simulink model "playback_data"  (R2015a)
settings: Solver=FixedStepDiscrete  SolverMode=SingleTasking  StartTime=76  StopTime=110  FixedStep=sample_time  RelTol=1e-3
undefined symbols (not defined in the file): A1_notch_f1, A2_notch_f1, A_kalman_swing_load, A_kalman_transverse, A_kalman_vertical, A_lpf_accelerometer, A_lpf_dtau, A_lpf_fourbar_angles, A_lpf_imu, A_lpf_lateral_angle, B1_lpf_accelerometer, B1_lpf_dtau, B1_lpf_fourbar_angles, B1_lpf_imu, B1_lpf_lateral_angle, B1_notch_f1, B2_lpf_accelerometer, B2_lpf_dtau, B2_lpf_fourbar_angles, B2_lpf_imu, B2_lpf_lateral_angle, B2_notch_f1, B_dx_versus_x0, B_kalman_swing_load, B_kalman_transverse, B_kalman_vertical, backwards_K_sag_of_t, backwards_P_sag_of_t, C_kalman_swing_load, C_kalman_transverse, C_kalman_vertical, com_leg_motor, com_torso, contact_threshold, control_start_time, d_ankle_to_foot, d_vertical_com, desired_com_forward_velocity, desired_com_lateral_velocity, desired_initial_leg_roll_left, desired_initial_leg_roll_right, desired_stance_beta2, desired_standing_torso_pitch, desired_standing_torso_roll, desired_standing_z, desired_torso_pitch, desired_torso_roll, Discrete, enable_bouncing, fcut_contact, fdesignblkfcn, forward_dx_of_dxstar, forward_x_of_dxstar, g, gcbh, HIP_MTR_MAX_CONT_TORQUE, HIP_MTR_MAX_TORQUE, i_leg_motor, i_robot, i_torso ... (+78)
libraries: simulink x65, dsparch4 x18, ctrlSharedLib x14, dspfdesign x4
(part 9 of 13)

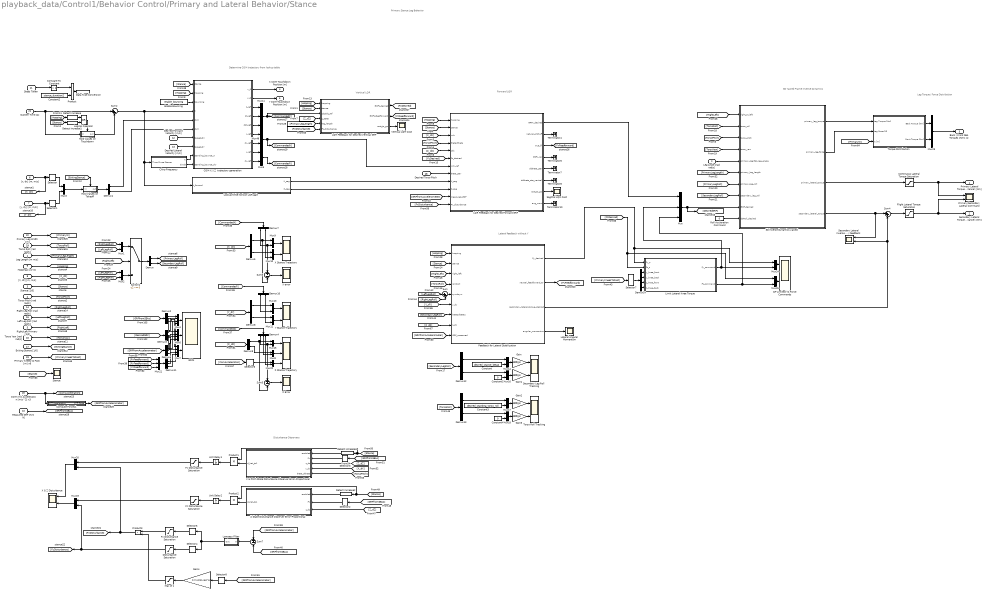
== system playback_data/Control1/Behavior Control/Primary and Lateral Behavior/Stance ==
  note: Lateral feedback without Y
  note: 3D Yawed Frame Inverse Dynamics
  note: Forward LQR
  note: Vertical LQR
  note: Determine COM trajectory
      | from lookup table
  note: Primary Stance Leg Behavior
  note: Disturbance Observers
  note: Leg Torque / Force
      | Distribution
  Leg Length [m m/s] : Inport
  Torso Pitch [rad rad/s] : Inport  Port=2
  Stance [1/0] : Inport  Port=3
  Leg Angle [rad rad/s] : Inport  Port=4
  Right/Left Primary [1/0] : Inport  Port=5
  "[x, dx] [m, m/s]" : Inport  Port=6
  "[y, dy] [m, m/s]" : Inport  Port=7
  "[z, dz] [m, m/s]" : Inport  Port=8
  Hopping [1 or 0] : Inport  Port=9
  Measured GRF [N N N] : Inport  Port=10
  Steps Taken : Inport  Port=11
  Desired Forward Velocity [m/s] : Inport  Port=12
  Desired Lateral Velocity [m/s] : Inport  Port=13
  Right Leg Roll [rad rad/s] : Inport  Port=14
  Left Leg Roll [rad rad/s] : Inport  Port=15
  Torso Yaw [rad rad/s] : Inport  Port=16
  Exiting Stance [1/0] : Inport  Port=17
  Desired Torso Pitch : Inport  Port=18
  Torso Roll [rad rad/s] : Inport  Port=19
  COM XYZ Acceleration [m/s^2] x3 : Inport  Port=20
  System Time [s] : Inport  Port=21
  Primary Leg Width [m] : Inport  Port=22
  Primary Knees to Foot [m] x6 : Inport  Port=23
  3D Inverse Dynamics yawed : MATLAB Function  TreatAsAtomicUnit=on
  COM X,Y,Z  trajectory generation : MATLAB Function  TreatAsAtomicUnit=on
  Chirp Frequency : Subsystem
  Compare To Constant : simulink/Logic and Bit Operations/Compare To Constant  relop=<  const=1  OutDataTypeStr=uint8
  Compute Forces1 : Subsystem
  Constant : Constant  Value=desired_stance_beta2
  Constant1 : Constant  Value=0
  Constant2 : Constant  Value=stance_duration/2
  Constant3 : Constant  Value=desired_standing_torso_roll
  Constant4 : Constant  Value=0
  Continuous Lateral Torque Saturation : Saturate  UpperLimit=max_primary_lateral_stance_torque  LowerLimit=-max_primary_lateral_stance_torque
      settings: AttributesFormatString=Top: %<UpperLimit>\nBottom: %<LowerLimit>
  Data Type Conversion : DataTypeConversion  OutDataTypeStr=double
  Demux{,1,5,7..10,12..13} (9 alike) : Demux  Outputs=2
  Demux{2..4,6,11} (5 alike) : Demux  Outputs=3
  Demux14 : Demux
  Detect Increase{,1..3} (4 alike) : simulink/Logic and Bit Operations/Detect Increase  vinit=0.0  InputProcessing=Inherited  OutDataTypeStr=boolean
  "Disturbance Saturation " : Saturate  UpperLimit=100  LowerLimit=-100
      settings: AttributesFormatString=Top: %<UpperLimit>\nBottom: %<LowerLimit>
  Enable Bouncing : Constant  Value=enable_bouncing  SampleTime=sample_time
  Feedback for Lateral Stabilization : MATLAB Function  TreatAsAtomicUnit=on
  Flight Lateral Torque Saturation : Saturate  UpperLimit=HIP_MTR_MAX_CONT_TORQUE  LowerLimit=-HIP_MTR_MAX_CONT_TORQUE
      settings: AttributesFormatString=Top: %<UpperLimit>\nBottom: %<LowerLimit>
  Fx Disturbance Saturation : Saturate  UpperLimit=100  LowerLimit=-100
      settings: AttributesFormatString=Top: %<UpperLimit>\nBottom: %<LowerLimit>
  "Fx Disturbance Saturation " : Saturate  UpperLimit=100  LowerLimit=-100
      settings: AttributesFormatString=Top: %<UpperLimit>\nBottom: %<LowerLimit>
  Fz Disturbance Saturation : Saturate  UpperLimit=100  LowerLimit=-100
      settings: AttributesFormatString=Top: %<UpperLimit>\nBottom: %<LowerLimit>
  GRFs : Scope  NumInputPorts=3
      settings: TimeRange=37.999  YMin=-1250~-2000~-1250  YMax=1500~3750~1750  SampleInput=on
  Gain{,1..3} (4 alike) : Gain  Gain=180/pi
  Gain4 : Gain  Gain=2/(m_total_real*g)
  Hold Values on Takeoff : Subsystem
  Hold Values on Touchdown : Subsystem
  LQR Feedback for Desired Forward GRF : MATLAB Function  TreatAsAtomicUnit=on
  LQR Feedback for Desired Vertical GRF : MATLAB Function  TreatAsAtomicUnit=on
  Lateral Angular Momentum : Scope
      settings: YMin=-3.5  YMax=4  SaveName=ScopeData20  SampleInput=on
  Limit Lateral Knee Torque : MATLAB Function  TreatAsAtomicUnit=on
  Logical Operator : Logic  Operator=OR  AllPortsSameDT=off  OutDataTypeStr=boolean
  Lookup finite horizon LQR gain : MATLAB Function  TreatAsAtomicUnit=on
  Lowpass Filter : Subsystem  DialogController=fdesignblkfcn  InitFcn=fdesignblkfcn(gcbh, {'InitFcn'});  mask(Lowpass Filter){}
      mask help: Design a lowpass filter
      settings: CopyFcn=fdesignblkfcn(gcbh, {'CopyFcn'});
      mask Help: helpview(mapfilelocation('dsp'), 'dsplowpassfilter');
      mask Display: disp('Lowpass')
  Max of 1 : Saturate  UpperLimit=1  LowerLimit=0
      settings: AttributesFormatString=Top: %<UpperLimit>\nBottom: %<LowerLimit>
  Mux : Mux  Inputs=3
  Mux{1..3,5,8..10,12..20,22..25,49} (21 alike) : Mux  Inputs=2
  Mux11 : Mux  Inputs=3
  Mux21 : Mux  Inputs=3
  Mux4 : Mux
  Mux6 : Mux
  Mux7 : Mux
  Primary/Secondary Lateral Command : Scope  NumInputPorts=2
      settings: YMin=40~-5  YMax=150~5  SaveName=ScopeData25  SampleInput=on
  Product{,1..3} (4 alike) : Product
  QP Limited YZ Force Commands : Scope  NumInputPorts=2
      settings: YMin=-200~0  YMax=30~700  SaveName=ScopeData26  SampleInput=on
  Roll Accleration Command : Constant  Value=0
  Sagittal LQR Cost : Scope
      settings: YMin=22.5  YMax=62.5  SaveName=ScopeData10  SampleInput=on
  Secondary Lateral Inverse Dynamics / Feedback : Scope  NumInputPorts=2
      settings: YMin=-3.5~-5  YMax=4~5  SaveName=ScopeData9  SampleInput=on
  Secondary Leg Roll Tracking : Scope  NumInputPorts=2
      settings: YMin=-3.5~-5  YMax=4~5  SaveName=ScopeData12  SampleInput=on
  Selector : Selector  InputPortWidth=2  Indices=[2]
  Selector1 : Selector  InputPortWidth=2  Indices=[2]
  Selector{2,4,6,8} (4 alike) : Selector  InputPortWidth=3  Indices=[3]
  Selector3 : Selector  InputPortWidth=3  Indices=[1]
  Selector5 : Selector  InputPortWidth=3  Indices=[1]
  Selector7 : Selector  InputPortWidth=6  Indices=[2 5 3 6]
  Stance : Scope
      settings: YMin=-0.05  YMax=0.11  SaveName=stance_time_history  SampleInput=on
  Sum : Sum  Inputs=|+-
  Sum2 : Sum  Inputs=|+-
  Sum4 : Sum  Inputs=|++
  Sum5 : Sum  Inputs=+-
  Sum6 : Sum  Inputs=+-
  Sum7 : Sum  Inputs=+-
  Switch1 : Switch  Criteria=u2 ~= 0
  Terminator{4,6..8,10} (5 alike) : Terminator
  Torque Distribution : Subsystem
  Torso Roll Tracking : Scope  NumInputPorts=2
      settings: YMin=-3.5~-5  YMax=4~5  SaveName=ScopeData15  SampleInput=on
  Unit Delay1 : UnitDelay  SampleTime=sample_time
  Unit Delay2 : UnitDelay  SampleTime=sample_time
  Vertical LQR Cost : Scope
      settings: YMin=11  YMax=16  SaveName=ScopeData18  SampleInput=on
  X & Pitch State Disturbance Observer Error-Proportional : MATLAB Function  TreatAsAtomicUnit=on
  X & Z Disturbance : Scope  NumInputPorts=2
      settings: YMin=-125~-800  YMax=175~700  SaveName=ScopeData16  SampleInput=on
  X Stance Trajectory : Scope  NumInputPorts=2
      settings: YMin=0~-0.02  YMax=0.005~0.03  SaveName=ScopeData8  SampleInput=on
  X error : Scope
      settings: YMin=-0.05  YMax=0.11  SaveName=ScopeData24  SampleInput=on
  Y Stance Trajectory : Scope  NumInputPorts=2
      settings: YMin=0.005~-0.5  YMax=0.1~0.3  SaveName=ScopeData5  SampleInput=on
  Z Error : Scope
      settings: YMin=-0.007  YMax=0.0005  SaveName=ScopeData23  SampleInput=on
  Z Stance Trajectory : Scope  NumInputPorts=3
      settings: YMin=0.85~-0.4~-3  YMax=0.98~0.6~11  SaveName=z_stance_trajectory  SampleInput=on
  Z State Disturbance Observer Error-Proportional : MATLAB Function  TreatAsAtomicUnit=on
  Primary Lateral Torque Command (stance) [Nm] : Outport
  Secondary Lateral Torque Command (stance) [Nm] : Outport  Port=2
  Back / Front SEA Torques [Nm] x2 : Outport  Port=3
  X COM Touchdown Position [m] : Outport  Port=4
  Y COM Touchdown Position [m] : Outport  Port=5
  wires:
  Fz Disturbance Saturation/1 -> Mux19/1
  Selector5/1 -> "Fx Disturbance Saturation "/1
  "Disturbance Saturation "/1 -> [FzDisturbance], Mux19/2
  Max of 1/1 -> Product3/2
  "Fx Disturbance Saturation "/1 -> Product3/1
  Gain4/1 -> Max of 1/1
  Selector8/1 -> Gain4/1
  [GRFfromAccelerometer] -> Selector8/1
  Limit Lateral Knee Torque/2(Fz_command) -> Mux/3, Mux25/2
  [FzDisturbance] -> LQR Feedback for Desired Vertical GRF/6(Fz_disturbance)
  [FxDisturbance] -> LQR Feedback for Desired Forward GRF/12(Fx_disturbance)
  Lowpass Filter/1(Out) -> Selector5/1, Selector4/1
  Chirp Frequency/2(dw/dt) -> COM X,Y,Z  trajectory generation/10(standing_bounce_dw)
  [Stance] -> Stance/1
  Chirp Frequency/1(w) -> COM X,Y,Z  trajectory generation/9(standing_bounce_w)
  Selector2/1 -> Z State Disturbance Observer Error-Proportional/2(Fz)
  Sum7/1 -> Lowpass Filter/1(In)
  Product3/1 -> Mux20/2, [FxDisturbance]
  Mux20/1 -> X & Z Disturbance/1
  [GRFfromAccelerometer] -> Sum7/1
  Sum6/1 -> X error/1
  Demux7/1 -> Mux9/2, Sum6/1
  Demux5/1 -> Mux9/1, Sum6/2
  Unit Delay2/1 -> Fz Disturbance Saturation/1
  Unit Delay1/1 -> Fx Disturbance Saturation/1
  Selector3/1 -> X & Pitch State Disturbance Observer Error-Proportional/2(Fx)
  Fx Disturbance Saturation/1 -> Mux20/1
  Enable Bouncing/1 -> COM X,Y,Z  trajectory generation/3(bouncing)
  [RightLeft] -> Feedback for Lateral Stabilization/3(right_left)
  Constant4/1 -> Mux18/2
  Mux18/1 -> Gain3/1
  Demux13/2 -> Mux18/1
  Constant3/1 -> Mux17/2
  Demux13/1 -> Mux17/1
  Mux17/1 -> Gain2/1
  Gain3/1 -> Torso Roll Tracking/2
  Gain2/1 -> Torso Roll Tracking/1
  [TorsoRoll] -> Demux13/1
  Constant1/1 -> Mux16/2
  Demux12/2 -> Mux16/1
  Mux16/1 -> Gain1/1
  Gain1/1 -> Secondary Leg Roll Tracking/2
  Gain/1 -> Secondary Leg Roll Tracking/1
  Constant/1 -> Mux14/2
  Demux12/1 -> Mux14/1
  Mux14/1 -> Gain/1
  [SecondaryLegRoll] -> Demux12/1
  Feedback for Lateral Stabilization/3(secondary_lateral_torque_desired) -> Sum4/2, Secondary Lateral Inverse Dynamics / Feedback/2
  Sum4/1 -> Flight Lateral Torque Saturation/1
  3D Inverse Dynamics yawed/3(primary_lateral_torque) -> Continuous Lateral Torque Saturation/1
  3D Inverse Dynamics yawed/4(secondary_lateral_torque) -> Secondary Lateral Inverse Dynamics / Feedback/1, Sum4/1
  Sum/1 -> Feedback for Lateral Stabilization/5(symdsym)
  [SecondaryLegRoll] -> Feedback for Lateral Stabilization/7(beta2dbeta2)
  [Y_dY] -> Feedback for Lateral Stabilization/6(y_dy)
  [RightLegRoll] -> Sum/2
  [LeftLegRoll] -> Sum/1
  Roll Accleration Command/1 -> 3D Inverse Dynamics yawed/10(ddRoll_desired)
  Feedback for Lateral Stabilization/1(Fy_desired) -> Limit Lateral Knee Torque/1(Fy_s), Mux24/1
  Continuous Lateral Torque Saturation/1 -> Primary/Secondary Lateral Command/1, Primary Lateral Torque Command (stance) [Nm]/1
  Demux11/3 -> Mux7/4
  Demux11/2 -> Mux6/4
  Demux11/1 -> Mux4/4
  Mux/1 -> [DesiredGRF], 3D Inverse Dynamics yawed/9(GRF_desired)
  LQR Feedback for Desired Forward GRF/1(GRFx_desired) -> Mux/1
  Left Leg Roll [rad rad/s]/1 -> [LeftLegRoll]
  Right/Left Primary [1/0]/1 -> [RightLeft]
  [CommandedY] -> Demux10/1
  [CommandedX] -> Demux7/1
  [Y_dY] -> Demux8/1
  Demux10/2 -> Mux12/2
  Demux10/1 -> Mux13/2
  Demux8/2 -> Mux12/1
  Demux8/1 -> Mux13/1
  Mux12/1 -> Y Stance Trajectory/2
  Mux13/1 -> Y Stance Trajectory/1
  [X_dX] -> Demux5/1
  Demux7/2 -> Mux10/2
  Demux5/2 -> Mux10/1
  Mux10/1 -> X Stance Trajectory/2
  Mux9/1 -> X Stance Trajectory/1
  Demux3/3 -> Mux7/2
  Demux3/2 -> Mux6/2
  Demux3/1 -> Mux4/2
  Demux2/3 -> Mux7/1
  Demux2/2 -> Mux6/1
  Mux7/1 -> GRFs/3
  Mux6/1 -> GRFs/2
  Demux2/1 -> Mux4/1
  Mux4/1 -> GRFs/1
  [DesiredGRF] -> Demux3/1
  [GRFfromSEAs] -> Demux2/1
  Torso Roll [rad rad/s]/1 -> [TorsoRoll]
  [PrimaryLegLength] -> LQR Feedback for Desired Vertical GRF/5(leg_length)
  Leg Length [m m/s]/1 -> [PrimaryLegLength]
  System Time [s]/1 -> Sum2/1, Hold Values on Touchdown/1(in)
  [GRFfromAccelerometer] -> Feedback for Lateral Stabilization/9(GRF_measured)
  [Hopping] -> Feedback for Lateral Stabilization/1(hopping)
  [ExitingStance] -> Hold Values on Takeoff/Trigger
  Exiting Stance [1/0]/1 -> [ExitingStance]
  Torso Yaw [rad rad/s]/1 -> [TorsoYaw]
  Desired Lateral Velocity [m/s]/1 -> COM X,Y,Z  trajectory generation/8(target_DY)
  Selector1/1 -> Mux3/2
  Hold Values on Takeoff/1(out) -> Demux1/1
  Mux3/1 -> Hold Values on Takeoff/1(in)
  "[y, dy] [m, m/s]"/1 -> Selector1/1, [Y_dY]
  [RightLeft] -> Switch1/2
  [RightLegRoll] -> Mux2/2
  [LeftLegRoll] -> Mux2/1
  [LeftLegRoll] -> Mux1/2
  [RightLegRoll] -> Mux1/1
  Right Leg Roll [rad rad/s]/1 -> [RightLegRoll]
  Mux2/1 -> Switch1/3
  Mux1/1 -> Switch1/1
  Demux/1 -> [PrimaryLegRoll]
  Demux/2 -> [SecondaryLegRoll]
  Switch1/1 -> Demux/1
  [PrimaryLegRoll] -> 3D Inverse Dynamics yawed/7(primary_leg_roll)
  [SecondaryLegRoll] -> 3D Inverse Dynamics yawed/8(secondary_leg_roll)
  Leg Angle [rad rad/s]/1 -> 3D Inverse Dynamics yawed/5(primary_sagittal_leg_angle)
  [PrimaryLegLength] -> 3D Inverse Dynamics yawed/6(primary_leg_length)
  [TorsoYaw] -> 3D Inverse Dynamics yawed/4(torso_yaw)
  [TorsoRoll] -> 3D Inverse Dynamics yawed/2(torso_roll)
  [TorsoPitch] -> 3D Inverse Dynamics yawed/3(torso_pitch)
  Mux5/1 -> [CommandedY]
  COM X,Y,Z  trajectory generation/2(y_0) -> Y COM Touchdown Position [m]/1
  [TorsoRoll] -> Feedback for Lateral Stabilization/4(rolldroll)
  [Stance] -> Feedback for Lateral Stabilization/2(stance)
  [Hopping] -> LQR Feedback for Desired Vertical GRF/1(hopping)
  Selector/1 -> Mux3/1
  Demux1/1 -> COM X,Y,Z  trajectory generation/5(dx0)
  [Stance] -> Detect Increase1/1
  [Hopping] -> Detect Increase/1
  Compare To Constant/1 -> Product/1
  Detect Increase1/1 -> Logical Operator/2
  Detect Increase/1 -> Logical Operator/1
  Constant2/1 -> Product/2
  Product/1 -> Data Type Conversion/1
  Steps Taken/1 -> Compare To Constant/1
  [GRFfromAccelerometer] -> LQR Feedback for Desired Forward GRF/11(measured_GRF)
  Measured GRF [N N N]/1 -> [GRFfromSEAs]
  [Hopping] -> LQR Feedback for Desired Forward GRF/1(hopping)
  [Hopping] -> COM X,Y,Z  trajectory generation/2(hopping)
  Hopping [1 or 0]/1 -> [Hopping]
  [RightLeft] -> 3D Inverse Dynamics yawed/1(right_or_left)
  Torso Pitch [rad rad/s]/1 -> [TorsoPitch]
  LQR Feedback for Desired Forward GRF/8(ang_mom) -> Terminator10/1
  LQR Feedback for Desired Forward GRF/7(cost_to_go) -> Sagittal LQR Cost/1
  LQR Feedback for Desired Forward GRF/6(ddtheta_star_neutral) -> Terminator8/1
  LQR Feedback for Desired Forward GRF/5(ddtheta_star) -> Terminator7/1
  LQR Feedback for Desired Vertical GRF/3(cost_to_go) -> Vertical LQR Cost/1
  Demux1/2 -> COM X,Y,Z  trajectory generation/6(dy0)
  "[x, dx] [m, m/s]"/1 -> Selector/1, [X_dX]
  Logical Operator/1 -> Hold Values on Touchdown/Trigger
  [Stance] -> LQR Feedback for Desired Vertical GRF/2(stance)
  Stance [1/0]/1 -> [Stance]
  Hold Values on Touchdown/1(out) -> Sum2/2
  LQR Feedback for Desired Vertical GRF/1(GRFz_desired) -> [FzDesired]
  Sum2/1 -> Chirp Frequency/1(Time Since Stance), Lookup finite horizon LQR gain/1(t_forward), COM X,Y,Z  trajectory generation/4(t)
  Desired Forward Velocity [m/s]/1 -> COM X,Y,Z  trajectory generation/7(target_DX)
  [Z_dZ] -> LQR Feedback for Desired Forward GRF/5(zdz)
  Lookup finite horizon LQR gain/1(K_sag) -> LQR Feedback for Desired Forward GRF/9(K_sag)
  Desired Torso Pitch/1 -> LQR Feedback for Desired Forward GRF/8(theta_star)
  Mux49/1 -> LQR Feedback for Desired Forward GRF/7(xdx_ref), [CommandedX]
  [TorsoPitch] -> LQR Feedback for Desired Forward GRF/4(thetadtheta)
  [X_dX] -> LQR Feedback for Desired Forward GRF/3(xdx)
  Mux11/1 -> LQR Feedback for Desired Vertical GRF/3(zdzddz_ref), [CommandedZ]
  COM X,Y,Z  trajectory generation/5(ddz_ref) -> Mux11/3
  COM X,Y,Z  trajectory generation/4(dz_ref) -> Mux11/2
  COM X,Y,Z  trajectory generation/1(x_0) -> X COM Touchdown Position [m]/1
  COM X,Y,Z  trajectory generation/9(dy_ref) -> Mux5/2
  COM X,Y,Z  trajectory generation/8(y_ref) -> Mux5/1
  COM X,Y,Z  trajectory generation/7(dx_ref) -> Mux49/2
  COM X,Y,Z  trajectory generation/6(x_ref) -> Mux49/1
  [Stance] -> LQR Feedback for Desired Forward GRF/2(stance)
  COM X,Y,Z  trajectory generation/3(z_ref) -> Mux11/1
  [Z_dZ] -> LQR Feedback for Desired Vertical GRF/4(z_state)
  Lookup finite horizon LQR gain/2(P_sag) -> LQR Feedback for Desired Forward GRF/10(P_sag)
  [Stance] -> COM X,Y,Z  trajectory generation/1(stance)
  LQR Feedback for Desired Forward GRF/4(GRFx_lqr) -> Terminator6/1
  Feedback for Lateral Stabilization/4(angular_momentum) -> Lateral Angular Momentum/1
  Demux6/1 -> Mux4/3
  Demux6/2 -> Mux6/3
  Demux6/3 -> Mux7/3
  Flight Lateral Torque Saturation/1 -> Primary/Secondary Lateral Command/2, Secondary Lateral Torque Command (stance) [Nm]/1
  "[z, dz] [m, m/s]"/1 -> [Z_dZ]
  [Z_dZ] -> X & Pitch State Disturbance Observer Error-Proportional/3(z_dz)
  [TorsoPitch] -> X & Pitch State Disturbance Observer Error-Proportional/5(theta_dtheta)
  [X_dX] -> X & Pitch State Disturbance Observer Error-Proportional/4(x_dx)
  [GRFfromSEAs] -> Selector3/1
  Detect Increase3/1 -> X & Pitch State Disturbance Observer Error-Proportional/1(enabled)
  Detect Increase2/1 -> Z State Disturbance Observer Error-Proportional/1(enabled)
  [GRFfromSEAs] -> Selector2/1
  [Z_dZ] -> Z State Disturbance Observer Error-Proportional/3(z_dz)
  Product1/1 -> Unit Delay1/1
  Product2/1 -> Unit Delay2/1
  X & Pitch State Disturbance Observer Error-Proportional/1(d_hat_tp1) -> Product1/2
  [Stance] -> Product1/1, Detect Increase3/1
  Z State Disturbance Observer Error-Proportional/1(d_hat_tp1) -> Product2/2
  [Stance] -> Product2/1, Detect Increase2/1
  Mux19/1 -> X & Z Disturbance/2
  [GRFfromSEAs] -> Sum7/2
  Selector4/1 -> "Disturbance Saturation "/1
  COM XYZ Acceleration [m/s^2] x3/1 -> Compute Forces1/1(XYZ Acceleration), [ComAcceleration]
  [GRFfromAccelerometer] -> Demux6/1
  LQR Feedback for Desired Vertical GRF/2(GRFz_feedforward) -> [FzFeedforward]
  Mux21/1 -> Demux11/1
  [FzFeedforward] -> Mux21/3
  Mux15/1 -> Z Stance Trajectory/1
  Mux8/1 -> Z Stance Trajectory/2
  [Z_dZ] -> Demux9/1
  Demux9/1 -> Mux15/1, Sum5/2
  Demux9/2 -> Mux8/1
  Demux4/1 -> Mux15/2, Sum5/1
  Demux4/2 -> Mux8/2
  Demux4/3 -> Mux22/2
  [CommandedZ] -> Demux4/1
  Sum5/1 -> Z Error/1
  Mux22/1 -> Z Stance Trajectory/3
  [ComAcceleration] -> Selector6/1
  Selector6/1 -> Mux22/1
  3D Inverse Dynamics yawed/1(primary_leg_torque) -> Torque Distribution/1(Leg Torque [Nm])
  [PrimaryW] -> Torque Distribution/3(w [m])
  3D Inverse Dynamics yawed/2(primary_leg_force) -> Torque Distribution/2(Leg Force [N])
  Primary Leg Width [m]/1 -> [PrimaryW]
  Torque Distribution/1(Back Torque [Nm]) -> Mux23/1
  Torque Distribution/2(Front Torque [Nm]) -> Mux23/2
  Mux23/1 -> Back / Front SEA Torques [Nm] x2/1
  [FxFeedforward] -> Mux21/1
  [FzDesired] -> LQR Feedback for Desired Forward GRF/6(Fz_desired)
  [FzDesired] -> Limit Lateral Knee Torque/2(Fz_s), Mux25/1
  [Z_dZ] -> Feedback for Lateral Stabilization/8(z_dz)
  [FyFeedforward] -> Mux21/2
  Compute Forces1/1(XYZ Force) -> [GRFfromAccelerometer]
  LQR Feedback for Desired Forward GRF/3(true_ff) -> [FxFeedforward]
  LQR Feedback for Desired Forward GRF/2(netural_pitch_ff) -> Terminator4/1
  Feedback for Lateral Stabilization/2(neutral_feedforward_Fy) -> [FyFeedforward]
  Primary Knees to Foot [m] x6/1 -> [PrimaryKneesToFoot]
  [PrimaryKneesToFoot] -> Selector7/1
  Demux14/1 -> Limit Lateral Knee Torque/3(y_knee_front)
  Demux14/2 -> Limit Lateral Knee Torque/4(y_knee_back)
  Demux14/3 -> Limit Lateral Knee Torque/5(z_knee_front)
  Demux14/4 -> Limit Lateral Knee Torque/6(z_knee_back)
  Selector7/1 -> Demux14/1
  Mux24/1 -> QP Limited YZ Force Commands/1
  Mux25/1 -> QP Limited YZ Force Commands/2
  Limit Lateral Knee Torque/1(Fy_command) -> Mux24/2, Mux/2

== system playback_data/Control1/Behavior Control/Secondary Leg Behavior/Back//Front PD ==
  Desired Position [rad] [back front] : Inport
  Desired Velocity [rad/s] [back front] : Inport  Port=2
  Measured Position [rad] [back front] : Inport  Port=3
  Measured Velocity [rad/s] [back front] : Inport  Port=4
  Back Tracking : Scope  NumInputPorts=2
      settings: YMin=3.725~-1  YMax=4.05~0.9  SaveName=ScopeData6  SampleInput=on
  Front Tracking : Scope  NumInputPorts=2
      settings: YMin=-1~-0.8  YMax=1~1.4  SaveName=ScopeData31  SampleInput=on
  Kp_SEA_Trajectory : Constant  Value=kp_velocity_swing_trajectory
  Mux{1..2,12..13} (4 alike) : Mux  Inputs=2
  Product1 : Product
  Selector{,1..3} (4 alike) : Selector  InputPortWidth=2  Indices=[1]
  Selector{4..7} (4 alike) : Selector  InputPortWidth=2  Indices=[2]
  Sum7 : Sum  Inputs=|+-
  Sum9 : Sum
  Commanded Velocity [rad/s] [back front] : Outport
  wires:
  Selector7/1 -> Mux1/2
  Selector6/1 -> Mux1/1
  Selector4/1 -> Mux2/1
  Selector5/1 -> Mux2/2
  Selector3/1 -> Mux12/2
  Selector2/1 -> Mux12/1
  Selector1/1 -> Mux13/2
  Selector/1 -> Mux13/1
  Mux2/1 -> Front Tracking/1
  Mux1/1 -> Front Tracking/2
  Desired Position [rad] [back front]/1 -> Sum7/1, Selector1/1, Selector5/1
  Mux13/1 -> Back Tracking/1
  Mux12/1 -> Back Tracking/2
  Product1/1 -> Sum9/1
  Sum7/1 -> Product1/1
  Measured Position [rad] [back front]/1 -> Sum7/2, Selector/1, Selector4/1
  Desired Velocity [rad/s] [back front]/1 -> Sum9/2, Selector2/1, Selector6/1
  Measured Velocity [rad/s] [back front]/1 -> Selector3/1, Selector7/1
  Sum9/1 -> Commanded Velocity [rad/s] [back front]/1
  Kp_SEA_Trajectory/1 -> Product1/2

== system playback_data/Control1/Behavior Control/Secondary Leg Behavior/Lowpass Filter (Swing) ==
  In : Inport
  Generated Filter Block : dsparch4/Biquad Filter  Tag=BlockMethodSubSystem  IIRFiltStruct=Direct form II  CoeffSource=Specify via dialog  BiQuadCoeffs=[1.0218648663828083 -2 1.0218648663828083 1 -1.9114378222117407 0.91557643487411833]  a0Flag=Warning  IC=0  ICnum=0  ICden=0  denAccumFracLength=30  denProdOutputFracLength=30  secondMemoryFracLength=15  roundingMode=Floor  overflowMode=off  ScaleValues=[0.0041174265739107223;22.985401576126357]  optimizeScaleValues=off  ScaleValueMode=Specify via input port (g)  scaleValueFracLength=14  FilterSource=Specify via dialog  FilterObject=Hm_biquad
  Out : Outport
  wires:
  Generated Filter Block/1 -> Out/1
  In/1 -> Generated Filter Block/1

== system playback_data/Control1/Behavior Control/State Estimation/Kalman Filtering ==
  "COM from Left Foot [body, yawed, global]" : Inport  SampleTime=sample_time
  "COM from Right Foot [body, yawed, global]" : Inport  Port=2  SampleTime=sample_time
  GRFx [N] : Inport  Port=3  SampleTime=sample_time
  GRFy [N] : Inport  Port=4  SampleTime=sample_time
  GRFz [N] : Inport  Port=5  SampleTime=sample_time
  Right Vertical GRF [N] : Inport  Port=6  SampleTime=sample_time
  Left Vertical GRF [N] : Inport  Port=7  SampleTime=sample_time
  "Initial [x, dx, ddx] [m, m/s, m/s^2]" : Inport  Port=8  PortDimensions=3  SampleTime=sample_time
  "Initial [y, dy, ddy] [m, m/s, m/s^2]" : Inport  Port=9  PortDimensions=3  SampleTime=sample_time
  "Initial [z, dz, ddz] [m m/s m/s^2]" : Inport  Port=10  PortDimensions=3  SampleTime=sample_time
  COM XYZ Acceleration [m/s^2] x3 : Inport  Port=11  SampleTime=sample_time
  Entering Stance [1/0] : Inport  Port=12  PortDimensions=1  SampleTime=sample_time
  Enable : EnablePort  StatesWhenEnabling=reset
  Difference : simulink/Discrete/Difference  ICPrevInput=0.0  InputProcessing=Inherited  OutMin=[]  OutMax=[]  OutDataType=fixdt(1, 16)  OutScaling=2^-10  DoSatur=off
  Difference1 : simulink/Discrete/Difference  ICPrevInput=0.0  InputProcessing=Inherited  OutMin=[]  OutMax=[]  OutDataType=fixdt(1, 16)  OutScaling=2^-10  DoSatur=off
  Difference2 : simulink/Discrete/Difference  ICPrevInput=0.0  InputProcessing=Inherited  OutMin=[]  OutMax=[]  OutDataType=fixdt(1, 16)  OutScaling=2^-10  DoSatur=off
  Logical Operator : Logic  Operator=NOT  AllPortsSameDT=off  OutDataTypeStr=boolean
  Measurement Noise Covariance Matricies : MATLAB Function  TreatAsAtomicUnit=on
  Mux : Mux  Inputs=3
  Mux1 : Mux  Inputs=3
  Mux3 : Mux  Inputs=3
  P0_kalman_transverse : Constant  Value=P0_kalman_transverse
  P0_kalman_transverse1 : Constant  Value=P0_kalman_transverse
  P0_kalman_vertical : Constant  Value=P0_kalman_vertical
  Product : Product
  Product1 : Product
  Product2 : Product
  X State Kalman Filter : ctrlSharedLib/Kalman Filter  TimeDomain=Discrete-Time  UseCurrentEstimator=on  ModelSource=Individual A, B, C, D matrices  ModelSourceVariable=A_kf  A=A_kalman_transverse  B=B_kalman_transverse  C=C_kalman_transverse  D=0  NumberOfStates=2  NumberOfInputs=1  NumberOfOutputs=2  InitialEstimateSource=Input port  X0=initial_dx_estimate  P0=P0_kalman_transverse  UseK=off  UseGH=on  NumberOfProcessNoiseInputs=1  G=G_kalman_transverse  TimeInvariantG=on  H=0  TimeInvariantH=on  Q=Q_kalman_GRF_difference  TimeInvariantQ=on  R=1  TimeInvariantR=off  N=0  TimeInvariantN=on  AddInputPort=on  AddEnablePort=off  ExternalReset=Rising  OutputEstimatedY=off  OutputP=on  Ts=sample_time
  Y State Kalman Filter : ctrlSharedLib/Kalman Filter  TimeDomain=Discrete-Time  UseCurrentEstimator=on  ModelSource=Individual A, B, C, D matrices  ModelSourceVariable=A_kf  A=A_kalman_transverse  B=B_kalman_transverse  C=C_kalman_transverse  D=0  NumberOfStates=2  NumberOfInputs=1  NumberOfOutputs=2  InitialEstimateSource=Input port  X0=initial_dy_estimate  P0=P0_kalman_transverse  UseK=off  UseGH=on  NumberOfProcessNoiseInputs=1  G=G_kalman_transverse  TimeInvariantG=on  H=0  TimeInvariantH=on  Q=Q_kalman_GRF_difference  TimeInvariantQ=on  R=1  TimeInvariantR=off  N=0  TimeInvariantN=on  AddInputPort=on  AddEnablePort=off  ExternalReset=Rising  OutputEstimatedY=off  OutputP=on  Ts=sample_time
  Z State Kalman Filter : ctrlSharedLib/Kalman Filter  TimeDomain=Discrete-Time  UseCurrentEstimator=on  ModelSource=Individual A, B, C, D matrices  ModelSourceVariable=A_kf  A=A_kalman_vertical  B=B_kalman_vertical  C=C_kalman_vertical  D=0  NumberOfStates=2  NumberOfInputs=1  NumberOfOutputs=2  InitialEstimateSource=Input port  X0=[initial_z_estimate; initial_dz_estimate]  P0=P0_kalman_vertical  UseK=off  UseGH=on  NumberOfProcessNoiseInputs=1  G=G_kalman_vertical  TimeInvariantG=on  H=0  TimeInvariantH=on  Q=Q_kalman_GRF_difference  TimeInvariantQ=on  R=1  TimeInvariantR=off  N=0  TimeInvariantN=on  AddInputPort=on  AddEnablePort=off  OutputEstimatedY=off  OutputP=on  Ts=sample_time
  eigen values : MATLAB Function  TreatAsAtomicUnit=on
  eigen values1 : MATLAB Function  TreatAsAtomicUnit=on
  eigen values2 : MATLAB Function  TreatAsAtomicUnit=on
  left x yawed : Selector  InputPortWidth=9  Indices=[4]
  left y yawed : Selector  InputPortWidth=9  Indices=[5]
  left z yawed : Selector  InputPortWidth=9  Indices=[6]
  right x yawed : Selector  InputPortWidth=9  Indices=[4]
  right y yawed : Selector  InputPortWidth=9  Indices=[5]
  right z yawed : Selector  InputPortWidth=9  Indices=[6]
  x acceleration : Selector  InputPortWidth=3  Indices=[1]
  y acceleration : Selector  InputPortWidth=3  Indices=[2]
  z acceleration : Selector  InputPortWidth=3  Indices=[3]
  "[x, dx, ddx] [m/s, m/s^2]" : Outport
  "[y, dy, ddy] [m/s, m/s^2]" : Outport  Port=2
  "[z, dz, ddz] [m, m/s, m/s^2]" : Outport  Port=3
  "[x, dx, ddx] uncertainty" : Outport  Port=4
  "[y, dy, ddy] uncertainty" : Outport  Port=5
  "[z, dz, ddz] uncertainty" : Outport  Port=6
  wires:
  GRFz [N]/1 -> Difference/1
  Product/1 -> Z State Kalman Filter/1
  Product1/1 -> Y State Kalman Filter/1
  Product2/1 -> X State Kalman Filter/1
  Difference2/1 -> Product2/2
  Difference1/1 -> Product1/2
  Entering Stance [1/0]/1 -> Logical Operator/1, X State Kalman Filter/5, Y State Kalman Filter/5
  Difference/1 -> Product/2
  Logical Operator/1 -> Product1/1, Product/1, Product2/1
  eigen values/1(E) -> "[z, dz, ddz] uncertainty"/1
  Z State Kalman Filter/2 -> eigen values/1(Z)
  Y State Kalman Filter/2 -> eigen values1/1(Z)
  X State Kalman Filter/2 -> eigen values2/1(Z)
  "Initial [z, dz, ddz] [m m/s m/s^2]"/1 -> Z State Kalman Filter/3
  P0_kalman_vertical/1 -> Z State Kalman Filter/4
  "Initial [y, dy, ddy] [m, m/s, m/s^2]"/1 -> Y State Kalman Filter/3
  P0_kalman_transverse1/1 -> Y State Kalman Filter/4
  "Initial [x, dx, ddx] [m, m/s, m/s^2]"/1 -> X State Kalman Filter/3
  P0_kalman_transverse/1 -> X State Kalman Filter/4
  right z yawed/1 -> Mux3/2
  left z yawed/1 -> Mux3/1
  right y yawed/1 -> Mux1/2
  left y yawed/1 -> Mux1/1
  right x yawed/1 -> Mux/2
  "COM from Right Foot [body, yawed, global]"/1 -> right x yawed/1, right y yawed/1, right z yawed/1
  left x yawed/1 -> Mux/1
  "COM from Left Foot [body, yawed, global]"/1 -> left x yawed/1, left y yawed/1, left z yawed/1
  Left Vertical GRF [N]/1 -> Measurement Noise Covariance Matricies/1(vertical_GRF_L)
  Right Vertical GRF [N]/1 -> Measurement Noise Covariance Matricies/2(vertical_GRF_R)
  Mux/1 -> X State Kalman Filter/2  "yawed [left x, right x, ddx]"
  Mux1/1 -> Y State Kalman Filter/2  "yawed [left y, right y, ddy]"
  Measurement Noise Covariance Matricies/1(R_transverse) -> Y State Kalman Filter/6, X State Kalman Filter/6
  Measurement Noise Covariance Matricies/2(R_vertical) -> Z State Kalman Filter/5
  GRFx [N]/1 -> Difference2/1
  Mux3/1 -> Z State Kalman Filter/2  "yawed [left z, right z, ddz]"
  GRFy [N]/1 -> Difference1/1
  Z State Kalman Filter/1 -> "[z, dz, ddz] [m, m/s, m/s^2]"/1
  COM XYZ Acceleration [m/s^2] x3/1 -> x acceleration/1, y acceleration/1, z acceleration/1
  z acceleration/1 -> Mux3/3
  x acceleration/1 -> Mux/3
  y acceleration/1 -> Mux1/3
  Y State Kalman Filter/1 -> "[y, dy, ddy] [m/s, m/s^2]"/1
  eigen values2/1(E) -> "[x, dx, ddx] uncertainty"/1
  eigen values1/1(E) -> "[y, dy, ddy] uncertainty"/1
  X State Kalman Filter/1 -> "[x, dx, ddx] [m/s, m/s^2]"/1

== system playback_data/Control1/Behavior Control/State Estimation/Lowpass Filter ==
  In : Inport
  Generated Filter Block : dsparch4/Biquad Filter  Tag=BlockMethodSubSystem  IIRFiltStruct=Direct form II  CoeffSource=Specify via dialog  BiQuadCoeffs=[1.0218648663828083 -2 1.0218648663828083 1 -1.9114378222117407 0.91557643487411833]  a0Flag=Warning  IC=0  ICnum=0  ICden=0  denAccumFracLength=30  denProdOutputFracLength=30  secondMemoryFracLength=15  roundingMode=Floor  overflowMode=off  ScaleValues=[0.0041174265739107223;22.985401576126357]  optimizeScaleValues=off  ScaleValueMode=Specify via input port (g)  scaleValueFracLength=14  FilterSource=Specify via dialog  FilterObject=Hm_biquad
  Out : Outport
  wires:
  Generated Filter Block/1 -> Out/1
  In/1 -> Generated Filter Block/1

== system playback_data/Control/Actuator Control with Torque SEA commands/Contact Velocities/Velocity on Contact/Subsystem ==
  in : Inport
  Enable : EnablePort
  out : Outport
  wires:
  in/1 -> out/1

== system playback_data/Control/Actuator Control with Torque SEA commands/Contact Velocities/Velocity on Contact1/Subsystem ==
  in : Inport
  Enable : EnablePort
  out : Outport
  wires:
  in/1 -> out/1

== system playback_data/Control/Actuator Control with Torque SEA commands/Contact Velocities/Velocity on Contact2/Subsystem ==
  in : Inport
  Enable : EnablePort
  out : Outport
  wires:
  in/1 -> out/1

== system playback_data/Control/Actuator Control with Torque SEA commands/Contact Velocities/Velocity on Contact3/Subsystem ==
  in : Inport
  Enable : EnablePort
  out : Outport
  wires:
  in/1 -> out/1

== system playback_data/Control/Actuator Control with Torque SEA commands/Timers/Time on Contact/Subsystem ==
  in : Inport
  Enable : EnablePort
  out : Outport
  wires:
  in/1 -> out/1

== system playback_data/Control/Actuator Control with Torque SEA commands/Timers/Time on Contact1/Subsystem ==
  in : Inport
  Enable : EnablePort
  out : Outport
  wires:
  in/1 -> out/1

== system playback_data/Control/Actuator Control with Torque SEA commands/Timers/Time on Contact2/Subsystem ==
  in : Inport
  Enable : EnablePort
  out : Outport
  wires:
  in/1 -> out/1

== system playback_data/Control/Actuator Control with Torque SEA commands/Timers/Time on Contact3/Subsystem ==
  in : Inport
  Enable : EnablePort
  out : Outport
  wires:
  in/1 -> out/1

== system playback_data/Control/Behavior Control/Primary and Lateral Behavior/Circular Buffer/Enabled on Touchdown ==
  In : Inport
  Enable : EnablePort
  Out : Outport
  wires:
  In/1 -> Out/1

== system playback_data/Control/Behavior Control/Primary and Lateral Behavior/Flight/Back//Front PD ==
  Desired Position [rad] [back front] : Inport
  Desired Velocity [rad/s] [back front] : Inport  Port=2
  Measured Position [rad] [back front] : Inport  Port=3
  Measured Velocity [rad/s] [back front] : Inport  Port=4
  Back Tracking : Scope  NumInputPorts=2
      settings: YMin=3.725~-1  YMax=4.05~0.9  SaveName=ScopeData6  SampleInput=on
  Front Tracking : Scope  NumInputPorts=2
      settings: YMin=-1~-0.8  YMax=1~1.4  SaveName=ScopeData31  SampleInput=on
  Kp_SEA_Trajectory : Constant  Value=kp_velocity_swing_trajectory
  Mux{1..2,12..13} (4 alike) : Mux  Inputs=2
  Product1 : Product
  Selector{,1..3} (4 alike) : Selector  InputPortWidth=2  Indices=[1]
  Selector{4..7} (4 alike) : Selector  InputPortWidth=2  Indices=[2]
  Sum7 : Sum  Inputs=|+-
  Sum9 : Sum
  Commanded Velocity [rad/s] [back front] : Outport
  wires:
  Selector7/1 -> Mux1/2
  Selector6/1 -> Mux1/1
  Selector4/1 -> Mux2/1
  Selector5/1 -> Mux2/2
  Selector3/1 -> Mux12/2
  Selector2/1 -> Mux12/1
  Selector1/1 -> Mux13/2
  Selector/1 -> Mux13/1
  Mux2/1 -> Front Tracking/1
  Mux1/1 -> Front Tracking/2
  Desired Position [rad] [back front]/1 -> Sum7/1, Selector1/1, Selector5/1
  Mux13/1 -> Back Tracking/1
  Mux12/1 -> Back Tracking/2
  Product1/1 -> Sum9/1
  Sum7/1 -> Product1/1
  Measured Position [rad] [back front]/1 -> Sum7/2, Selector/1, Selector4/1
  Desired Velocity [rad/s] [back front]/1 -> Sum9/2, Selector2/1, Selector6/1
  Measured Velocity [rad/s] [back front]/1 -> Selector3/1, Selector7/1
  Sum9/1 -> Commanded Velocity [rad/s] [back front]/1
  Kp_SEA_Trajectory/1 -> Product1/2

== system playback_data/Control/Behavior Control/Primary and Lateral Behavior/Flight/Hold Values on Takeoff ==
  in : Inport
  Trigger : TriggerPort  ShowOutputPort=on  PortDimensions=1
  Subsystem : Subsystem
  out : Outport
  wires:
  Trigger/1 -> Subsystem/Enable
  Subsystem/1(out) -> out/1
  in/1 -> Subsystem/1(in)

== system playback_data/Control/Behavior Control/Primary and Lateral Behavior/Stance/Chirp Frequency ==
  Time Since Stance : Inport
  Chirp Freq Factor Saturation : Saturate  UpperLimit=standing_bounce_max_chirp_scale  LowerLimit=0
      settings: AttributesFormatString=Top: %<UpperLimit>\nBottom: %<LowerLimit>
  Compare To Constant1 : simulink/Logic and Bit Operations/Compare To Constant  relop=~=  const=standing_bounce_max_chirp_scale  OutDataTypeStr=boolean
  Constant1 : Constant
  Constant5 : Constant  Value=standing_bounce_increase_rate
  Product{1..4} (4 alike) : Product
  Sum : Sum  Inputs=++|
  standing_bounce_frequency : Constant  Value=standing_bounce_frequency
  w : Outport
  dw/dt : Outport  Port=2
  wires:
  Constant1/1 -> Sum/1
  Product4/1 -> Sum/2
  Sum/1 -> Chirp Freq Factor Saturation/1
  Time Since Stance/1 -> Product4/1
  Constant5/1 -> Product4/2, Product2/2
  Product2/1 -> Product1/2
  Compare To Constant1/1 -> Product1/1
  Product1/1 -> dw/dt/1
  Product3/1 -> w/1
  Chirp Freq Factor Saturation/1 -> Compare To Constant1/1, Product3/2
  standing_bounce_frequency/1 -> Product3/1, Product2/1

== system playback_data/Control/Behavior Control/Primary and Lateral Behavior/Stance/Compute Forces1 ==
  XYZ Acceleration : Inport
  Constant5 : Constant  Value=g
  Demux : Demux  Outputs=3
  Gain4 : Gain  Gain=m_total_real
  Mux : Mux  Inputs=3
  Sum8 : Sum  Inputs=|++
  XYZ Force : Outport
  wires:
  Demux/1 -> Mux/1
  Demux/2 -> Mux/2
  Demux/3 -> Sum8/1
  Sum8/1 -> Mux/3
  Mux/1 -> Gain4/1
  Gain4/1 -> XYZ Force/1
  XYZ Acceleration/1 -> Demux/1
  Constant5/1 -> Sum8/2

== system playback_data/Control/Behavior Control/Primary and Lateral Behavior/Stance/Hold Values on Takeoff ==
  in : Inport
  Trigger : TriggerPort  ShowOutputPort=on  PortDimensions=1
  Subsystem : Subsystem
  out : Outport
  wires:
  in/1 -> Subsystem/1(in)
  Subsystem/1(out) -> out/1
  Trigger/1 -> Subsystem/Enable

== system playback_data/Control/Behavior Control/Primary and Lateral Behavior/Stance/Hold Values on Touchdown ==
  in : Inport
  Trigger : TriggerPort  ShowOutputPort=on  PortDimensions=1
  Subsystem : Subsystem
  out : Outport
  wires:
  Trigger/1 -> Subsystem/Enable
  Subsystem/1(out) -> out/1
  in/1 -> Subsystem/1(in)

== system playback_data/Control/Behavior Control/Primary and Lateral Behavior/Stance/Lowpass Filter ==
  In : Inport
  Generated Filter Block : dsparch4/Biquad Filter  Tag=BlockMethodSubSystem  IIRFiltStruct=Direct form II  CoeffSource=Specify via dialog  BiQuadCoeffs=[1.2169083457291219 -2 1.2169083457291219 1 -1.7334293610249598 0.76768521888208641]  a0Flag=Warning  IC=0  ICnum=0  ICden=0  denAccumFracLength=30  denProdOutputFracLength=30  secondMemoryFracLength=15  roundingMode=Floor  overflowMode=off  ScaleValues=[0.034049223021428709;2.3191101889079508]  optimizeScaleValues=off  ScaleValueMode=Specify via input port (g)  scaleValueFracLength=14  FilterSource=Specify via dialog  FilterObject=Hm_biquad
  Out : Outport
  wires:
  Generated Filter Block/1 -> Out/1
  In/1 -> Generated Filter Block/1

== system playback_data/Control/Behavior Control/Primary and Lateral Behavior/Stance/Torque Distribution ==
  Leg Torque [Nm] : Inport
  Leg Force [N] : Inport  Port=2
  w [m] : Inport  Port=3
  Gain : Gain  Gain=0.5
  Gain1 : Gain  Gain=0.5
  Motor Torque Saturation Optimization : MATLAB Function  TreatAsAtomicUnit=on
  Product : Product  RndMeth=Zero
  Sum : Sum  Inputs=|++
  Sum1 : Sum  Inputs=+-|
  Back Torque [Nm] : Outport
  Front Torque [Nm] : Outport  Port=2
  wires:
  Sum1/1 -> Back Torque [Nm]/1
  Leg Torque [Nm]/1 -> Gain/1
  Sum/1 -> Front Torque [Nm]/1
  Motor Torque Saturation Optimization/1(t1) -> Sum/1, Sum1/1
  w [m]/1 -> Product/2
  Motor Torque Saturation Optimization/2(t2) -> Sum1/2, Sum/2
  Leg Force [N]/1 -> Product/1
  Product/1 -> Gain1/1
  Gain1/1 -> Motor Torque Saturation Optimization/2(x2s)
  Gain/1 -> Motor Torque Saturation Optimization/1(x1s)

== system playback_data/Control1/Actuator Control with Torque SEA commands/Contact Velocities/Velocity on Contact/Subsystem ==
  in : Inport
  Enable : EnablePort
  out : Outport
  wires:
  in/1 -> out/1

== system playback_data/Control1/Actuator Control with Torque SEA commands/Contact Velocities/Velocity on Contact1/Subsystem ==
  in : Inport
  Enable : EnablePort
  out : Outport
  wires:
  in/1 -> out/1

== system playback_data/Control1/Actuator Control with Torque SEA commands/Contact Velocities/Velocity on Contact2/Subsystem ==
  in : Inport
  Enable : EnablePort
  out : Outport
  wires:
  in/1 -> out/1

== system playback_data/Control1/Actuator Control with Torque SEA commands/Contact Velocities/Velocity on Contact3/Subsystem ==
  in : Inport
  Enable : EnablePort
  out : Outport
  wires:
  in/1 -> out/1

== system playback_data/Control1/Actuator Control with Torque SEA commands/Timers/Time on Contact/Subsystem ==
  in : Inport
  Enable : EnablePort
  out : Outport
  wires:
  in/1 -> out/1

== system playback_data/Control1/Actuator Control with Torque SEA commands/Timers/Time on Contact1/Subsystem ==
  in : Inport
  Enable : EnablePort
  out : Outport
  wires:
  in/1 -> out/1

== system playback_data/Control1/Actuator Control with Torque SEA commands/Timers/Time on Contact2/Subsystem ==
  in : Inport
  Enable : EnablePort
  out : Outport
  wires:
  in/1 -> out/1

== system playback_data/Control1/Actuator Control with Torque SEA commands/Timers/Time on Contact3/Subsystem ==
  in : Inport
  Enable : EnablePort
  out : Outport
  wires:
  in/1 -> out/1

== system playback_data/Control1/Behavior Control/Primary and Lateral Behavior/Circular Buffer/Enabled on Touchdown ==
  In : Inport
  Enable : EnablePort
  Out : Outport
  wires:
  In/1 -> Out/1

== system playback_data/Control1/Behavior Control/Primary and Lateral Behavior/Flight/Back//Front PD ==
  Desired Position [rad] [back front] : Inport
  Desired Velocity [rad/s] [back front] : Inport  Port=2
  Measured Position [rad] [back front] : Inport  Port=3
  Measured Velocity [rad/s] [back front] : Inport  Port=4
  Back Tracking : Scope  NumInputPorts=2
      settings: YMin=3.725~-1  YMax=4.05~0.9  SaveName=ScopeData6  SampleInput=on
  Front Tracking : Scope  NumInputPorts=2
      settings: YMin=-1~-0.8  YMax=1~1.4  SaveName=ScopeData31  SampleInput=on
  Kp_SEA_Trajectory : Constant  Value=kp_velocity_swing_trajectory
  Mux{1..2,12..13} (4 alike) : Mux  Inputs=2
  Product1 : Product
  Selector{,1..3} (4 alike) : Selector  InputPortWidth=2  Indices=[1]
  Selector{4..7} (4 alike) : Selector  InputPortWidth=2  Indices=[2]
  Sum7 : Sum  Inputs=|+-
  Sum9 : Sum
  Commanded Velocity [rad/s] [back front] : Outport
  wires:
  Selector7/1 -> Mux1/2
  Selector6/1 -> Mux1/1
  Selector4/1 -> Mux2/1
  Selector5/1 -> Mux2/2
  Selector3/1 -> Mux12/2
  Selector2/1 -> Mux12/1
  Selector1/1 -> Mux13/2
  Selector/1 -> Mux13/1
  Mux2/1 -> Front Tracking/1
  Mux1/1 -> Front Tracking/2
  Desired Position [rad] [back front]/1 -> Sum7/1, Selector1/1, Selector5/1
  Mux13/1 -> Back Tracking/1
  Mux12/1 -> Back Tracking/2
  Product1/1 -> Sum9/1
  Sum7/1 -> Product1/1
  Measured Position [rad] [back front]/1 -> Sum7/2, Selector/1, Selector4/1
  Desired Velocity [rad/s] [back front]/1 -> Sum9/2, Selector2/1, Selector6/1
  Measured Velocity [rad/s] [back front]/1 -> Selector3/1, Selector7/1
  Sum9/1 -> Commanded Velocity [rad/s] [back front]/1
  Kp_SEA_Trajectory/1 -> Product1/2

== system playback_data/Control1/Behavior Control/Primary and Lateral Behavior/Flight/Hold Values on Takeoff ==
  in : Inport
  Trigger : TriggerPort  ShowOutputPort=on  PortDimensions=1
  Subsystem : Subsystem
  out : Outport
  wires:
  Trigger/1 -> Subsystem/Enable
  Subsystem/1(out) -> out/1
  in/1 -> Subsystem/1(in)

== system playback_data/Control1/Behavior Control/Primary and Lateral Behavior/Stance/Chirp Frequency ==
  Time Since Stance : Inport
  Chirp Freq Factor Saturation : Saturate  UpperLimit=standing_bounce_max_chirp_scale  LowerLimit=0
      settings: AttributesFormatString=Top: %<UpperLimit>\nBottom: %<LowerLimit>
  Compare To Constant1 : simulink/Logic and Bit Operations/Compare To Constant  relop=~=  const=standing_bounce_max_chirp_scale  OutDataTypeStr=boolean
  Constant1 : Constant
  Constant5 : Constant  Value=standing_bounce_increase_rate
  Product{1..4} (4 alike) : Product
  Sum : Sum  Inputs=++|
  standing_bounce_frequency : Constant  Value=standing_bounce_frequency
  w : Outport
  dw/dt : Outport  Port=2
  wires:
  Constant1/1 -> Sum/1
  Product4/1 -> Sum/2
  Sum/1 -> Chirp Freq Factor Saturation/1
  Time Since Stance/1 -> Product4/1
  Constant5/1 -> Product4/2, Product2/2
  Product2/1 -> Product1/2
  Compare To Constant1/1 -> Product1/1
  Product1/1 -> dw/dt/1
  Product3/1 -> w/1
  Chirp Freq Factor Saturation/1 -> Compare To Constant1/1, Product3/2
  standing_bounce_frequency/1 -> Product3/1, Product2/1

== system playback_data/Control1/Behavior Control/Primary and Lateral Behavior/Stance/Compute Forces1 ==
  XYZ Acceleration : Inport
  Constant5 : Constant  Value=g
  Demux : Demux  Outputs=3
  Gain4 : Gain  Gain=m_total_real
  Mux : Mux  Inputs=3
  Sum8 : Sum  Inputs=|++
  XYZ Force : Outport
  wires:
  Demux/1 -> Mux/1
  Demux/2 -> Mux/2
  Demux/3 -> Sum8/1
  Sum8/1 -> Mux/3
  Mux/1 -> Gain4/1
  Gain4/1 -> XYZ Force/1
  XYZ Acceleration/1 -> Demux/1
  Constant5/1 -> Sum8/2

== system playback_data/Control1/Behavior Control/Primary and Lateral Behavior/Stance/Hold Values on Takeoff ==
  in : Inport
  Trigger : TriggerPort  ShowOutputPort=on  PortDimensions=1
  Subsystem : Subsystem
  out : Outport
  wires:
  in/1 -> Subsystem/1(in)
  Subsystem/1(out) -> out/1
  Trigger/1 -> Subsystem/Enable

== system playback_data/Control1/Behavior Control/Primary and Lateral Behavior/Stance/Hold Values on Touchdown ==
  in : Inport
  Trigger : TriggerPort  ShowOutputPort=on  PortDimensions=1
  Subsystem : Subsystem
  out : Outport
  wires:
  Trigger/1 -> Subsystem/Enable
  Subsystem/1(out) -> out/1
  in/1 -> Subsystem/1(in)

== system playback_data/Control1/Behavior Control/Primary and Lateral Behavior/Stance/Lowpass Filter ==
  In : Inport
  Generated Filter Block : dsparch4/Biquad Filter  Tag=BlockMethodSubSystem  IIRFiltStruct=Direct form II  CoeffSource=Specify via dialog  BiQuadCoeffs=[1.2169083457291219 -2 1.2169083457291219 1 -1.7334293610249598 0.76768521888208641]  a0Flag=Warning  IC=0  ICnum=0  ICden=0  denAccumFracLength=30  denProdOutputFracLength=30  secondMemoryFracLength=15  roundingMode=Floor  overflowMode=off  ScaleValues=[0.034049223021428709;2.3191101889079508]  optimizeScaleValues=off  ScaleValueMode=Specify via input port (g)  scaleValueFracLength=14  FilterSource=Specify via dialog  FilterObject=Hm_biquad
  Out : Outport
  wires:
  Generated Filter Block/1 -> Out/1
  In/1 -> Generated Filter Block/1

== system playback_data/Control1/Behavior Control/Primary and Lateral Behavior/Stance/Torque Distribution ==
  Leg Torque [Nm] : Inport
  Leg Force [N] : Inport  Port=2
  w [m] : Inport  Port=3
  Gain : Gain  Gain=0.5
  Gain1 : Gain  Gain=0.5
  Motor Torque Saturation Optimization : MATLAB Function  TreatAsAtomicUnit=on
  Product : Product  RndMeth=Zero
  Sum : Sum  Inputs=|++
  Sum1 : Sum  Inputs=+-|
  Back Torque [Nm] : Outport
  Front Torque [Nm] : Outport  Port=2
  wires:
  Sum1/1 -> Back Torque [Nm]/1
  Leg Torque [Nm]/1 -> Gain/1
  Sum/1 -> Front Torque [Nm]/1
  Motor Torque Saturation Optimization/1(t1) -> Sum/1, Sum1/1
  w [m]/1 -> Product/2
  Motor Torque Saturation Optimization/2(t2) -> Sum1/2, Sum/2
  Leg Force [N]/1 -> Product/1
  Product/1 -> Gain1/1
  Gain1/1 -> Motor Torque Saturation Optimization/2(x2s)
  Gain/1 -> Motor Torque Saturation Optimization/1(x1s)

== system playback_data/Control/Behavior Control/Primary and Lateral Behavior/Flight/Hold Values on Takeoff/Subsystem ==
  in : Inport
  Enable : EnablePort
  out : Outport
  wires:
  in/1 -> out/1

== system playback_data/Control/Behavior Control/Primary and Lateral Behavior/Stance/Hold Values on Takeoff/Subsystem ==
  in : Inport
  Enable : EnablePort
  out : Outport
  wires:
  in/1 -> out/1

== system playback_data/Control/Behavior Control/Primary and Lateral Behavior/Stance/Hold Values on Touchdown/Subsystem ==
  in : Inport
  Enable : EnablePort
  out : Outport
  wires:
  in/1 -> out/1

== system playback_data/Control1/Behavior Control/Primary and Lateral Behavior/Flight/Hold Values on Takeoff/Subsystem ==
  in : Inport
  Enable : EnablePort
  out : Outport
  wires:
  in/1 -> out/1

== system playback_data/Control1/Behavior Control/Primary and Lateral Behavior/Stance/Hold Values on Takeoff/Subsystem ==
  in : Inport
  Enable : EnablePort
  out : Outport
  wires:
  in/1 -> out/1

== system playback_data/Control1/Behavior Control/Primary and Lateral Behavior/Stance/Hold Values on Touchdown/Subsystem ==
  in : Inport
  Enable : EnablePort
  out : Outport
  wires:
  in/1 -> out/1

== matlab function playback_data/Control1/Actuator Control with Torque SEA commands/Detect Collision ==
  data: time input; spring_torque input; load_torque_derivative input; in_collision output; swing_collision_wait_time parameter
function in_collision = detect_collision(time, spring_torque, load_torque_derivative, swing_collision_wait_time)
    
    persistent collision_state time_of_collision;
    if isempty(collision_state)
        collision_state = logical(zeros(4,1));
        time_of_collision = zeros(4,1);
    end

    collision_detected = (abs(load_torque_derivative) > 2000 | abs(spring_torque) >= 50) & (time - time_of_collision > (1.5*swing_collision_wait_time));
    time_of_collision(collision_detected) = time;
    collision_state = collision_state | collision_detected;
    time_since_collision = time - time_of_collision;
    out_of_collision = (time_since_collision > swing_collision_wait_time) & (abs(spring_torque) < 50);
    collision_state(out_of_collision) = 0;
    %in_collision = collision_state;
    in_collision = [collision_state(1) | collision_state(2);
                    collision_state(1) | collision_state(2);
                    collision_state(3) | collision_state(4);
                    collision_state(3) | collision_state(4)];
    
end
